simulink model "simul_exp3"  (R2018a)
settings: Solver=VariableStepDiscrete  StartTime=0.0  StopTime=0.2  RelTol=1e-3
libraries: powerlib_meascontrol x12, powerlib x8
settings Model: Creator=PSA LAB  LastModifiedBy=PSA LAB

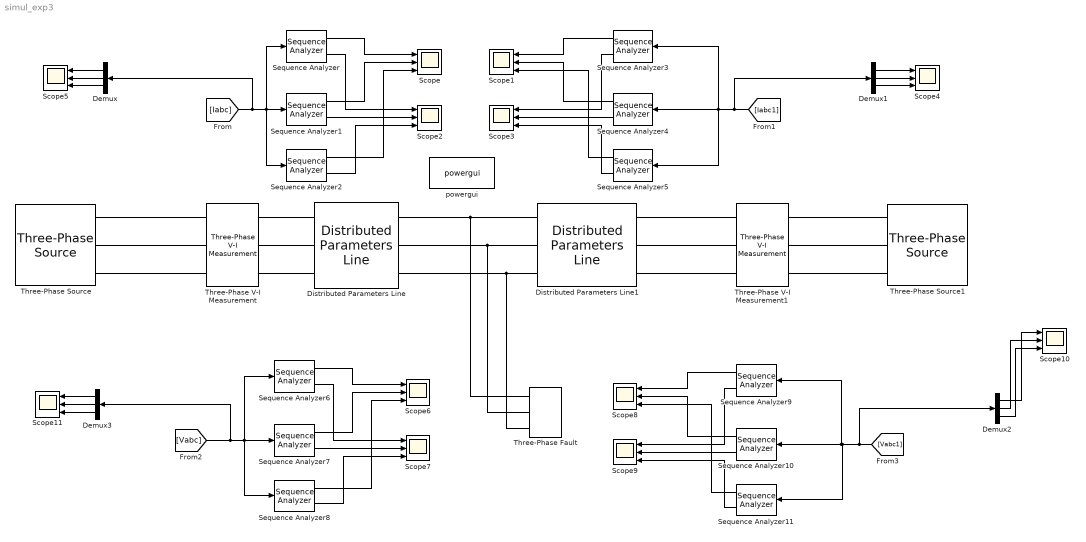
== system simul_exp3 ==
  Demux{,1..3} (4 alike) : Demux  Outputs=3
  Distributed Parameters Line : powerlib/Elements/Distributed Parameters Line  Phases=3  Frequency=50  Resistance=[0.0168 0.242]  Inductance=[0.223 0.724]/(2*pi*50)  Capacitance=[12.74e-9 7.751e-9]  Length=50  x1=[-0.00025 -1.56487866400999e-10 0 0;-0.0002 -1.54369226650682e-10 255080.19880985 -307468.607575482;-0.00015 -1.52212498603565e-10 259878.237181357 -303424.050313729;-0.0001 -1.50018214400022e-10 264612.154486481 -299304.627707794;-5e-05 -1.47786915446847e-10 269280.782701962 -295111.356163562]  x2=[-0.00025 -1.7683899889414e-10 0 0;-0.0002 -1.82309191569534e-10 234319.785127672 -322361.576827908;-0.00015 -1.87734402179861e-10 239354.313253658 -318641.272662729;-0.0001 -1.93113292135579e-10 244329.784284384 -314842.348531452;-5e-05 -1.98444534276079e-10 249244.970596823 -310965.741761762]  x3=[-0.00025 1.20606379414602e-11 0 0;-0.0002 1.20492587104112e-11 -418.457428681975 424.341761235616;-0.00015 1.20349065050724e-11 -425.071075319853 417.716567631808;-0.0001 1.20175848666357e-11 -431.579842030371 410.988308715365;-5e-05 1.1997298068956e-11 -437.982122872735 404.158644583495]  x4=[-0.00025 -1.34129195403542e-11 0 0;-0.0002 -1.33002997678989e-11 2423.35362344846 -3134.39626162489;-0.00015 -1.31843983454925e-11 2472.2876169882 -3095.94519461435;-0.0001 -1.30652438700767e-11 2520.61161055209 -3056.73024945266;-5e-05 -1.29428657412354e-11 2568.31368091779 -3016.76110184075]  x5=0.000211321273641276  V1=[1.455e-10 3.995e+05 3.995e+05;314.2 314.2 314.2;0.5771 0.7081 -0.8627]  V2=[5.043e-10 3.985e+05 3.985e+05;314.2 314.2 314.2;-0.8314 0.6441 -0.9267]  I1=[1.151e-11 596 596;314.2 314.2 314.2;-2.267 -2.348 2.365]  I2=[1.656e-11 3962 3962;314.2 314.2 314.2;0.6614 0.6737 -0.897]  nHarmo=1  Measurements=None
      settings: SourceProductName=Simscape Power Systems
  Distributed Parameters Line1 : powerlib/Elements/Distributed Parameters Line  Phases=3  Frequency=50  Resistance=[0.0168 0.242]  Inductance=[0.223 0.724]/(2*pi*50)  Capacitance=[12.74e-9 7.751e-9]  Length=100  x1=[-0.00045 -1.70021553368224e-10 208305.257615079 -339752.362121545;-0.0004 -1.77191466076833e-10 213616.157671673 -336438.5309367;-0.00035 -1.84317659442561e-10 218874.35113777 -333041.688578584;-0.0003 -1.91398375183826e-10 224078.54063281 -329562.67316722;-0.00025 -1.98431866239969e-10 229227.442100909 -326002.343097605;-0.0002 -2.05416397202318e-10 234319.785127672 -322361.576827908;-0.00015 -2.12350244742368e-10 239354.313253658 -318641.272662729;-0.0001 -2.19231698036993e-10 244329.784284384 -314842.348531452;-5e-05 -2.26059059190562e-10 249244.970596823 -310965.741761762]  x2=[-0.00045 -1.06944269874296e-10 163412.8471615 -363782.763094215;-0.0004 -1.04861400083317e-10 169106.738616573 -361171.106674324;-0.00035 -1.02752657310943e-10 174758.90551429 -358470.33668818;-0.0003 -1.00618561857898e-10 180367.953267046 -355681.119510365;-0.00025 -9.84596402803031e-11 185932.497926236 -352804.143338482;-0.0002 -9.62764252597519e-11 191451.166523731 -349840.118023352;-0.00015 -9.40694554718829e-11 196922.597410631 -346789.774893869;-0.0001 -9.18392754534677e-11 202345.440593236 -343653.866576558;-5e-05 -8.9586435468055e-11 207718.358066135 -340433.166809873]  x3=[-0.00045 -7.36346410085895e-12 -409.538920507377 443.963253695975;-0.0004 -7.37107802688559e-12 -416.461868407682 437.475725275183;-0.00035 -7.3768732497049e-12 -423.282060573609 430.880256265269;-0.0003 -7.38084833943238e-12 -429.997814224796 424.178473999522;-0.00025 -7.38300231527411e-12 -436.607472349517 417.372032042433;-0.0002 -7.38333464576877e-12 -443.109404113535 410.46260978171;-0.00015 -7.3818452489188e-12 -449.502005262476 403.451912013908;-0.0001 -7.37853449221059e-12 -455.783698517661 396.341668523796;-5e-05 -7.3734031925238e-12 -461.952933965275 389.133633657564]  x4=[-0.00045 5.90981358690036e-12 1835.53978451295 -3482.79405347785;-0.0004 5.8270331277052e-12 1890.01868985462 -3453.53298398477;-0.00035 5.74281493527755e-12 1944.03126136552 -3423.41980690421;-0.0003 5.6571797891962e-12 1997.56417225185 -3392.46195221203;-0.00025 5.57014881865206e-12 2050.60421406887 -3360.66705829565;-0.0002 5.48174349723485e-12 2103.13829997991 -3328.04297006936;-0.00015 5.39198563763478e-12 2155.15346798537 -3294.59773703879;-0.0001 5.30089738626064e-12 2206.63688412086 -3260.33961131473;-5e-05 5.20850121777547e-12 2257.57584562381 -3225.27704557708]  x5=0.000422642547282553  V1=[5.043e-10 3.985e+05 3.985e+05;314.2 314.2 314.2;-0.8978 0.5969 -0.9739]  V2=[1.841e-10 3.988e+05 3.988e+05;314.2 314.2 314.2;0.189 0.4691 -1.102]  I1=[3.598e-12 604 604;314.2 314.2 314.2;0.6362 -2.35 2.363]  I2=[5.12e-12 3937 3937;314.2 314.2 314.2;-2.674 0.5319 -1.039]  nHarmo=1  Measurements=None
      settings: SourceProductName=Simscape Power Systems
  Scope{,1..11} (12 alike) : Scope  NumInputPorts=3
  Sequence Analyzer{,3,6,9} (4 alike) : powerlib_meascontrol/Measurements/Sequence Analyzer  Freq=50  n=1  seq=Positive  InInit=[1, 0]  Ts=0
      settings: SourceProductName=Simscape Power Systems  SourceProductBaseCode=PS
  Sequence Analyzer{1,4,7,10} (4 alike) : powerlib_meascontrol/Measurements/Sequence Analyzer  Freq=50  n=1  seq=Negative  InInit=[1, 0]  Ts=0
      settings: SourceProductName=Simscape Power Systems  SourceProductBaseCode=PS
  Sequence Analyzer{2,5,8,11} (4 alike) : powerlib_meascontrol/Measurements/Sequence Analyzer  Freq=50  n=1  seq=Zero  InInit=[1, 0]  Ts=0
      settings: SourceProductName=Simscape Power Systems  SourceProductBaseCode=PS
  Three-Phase V-I Measurement : powerlib/Measurements/Three-Phase V-I Measurement  VoltageMeasurement=phase-to-phase  SetLabelV=on  LabelV=Vabc  Vpu=off  VpuLL=on  CurrentMeasurement=yes  SetLabelI=on  LabelI=Iabc  Ipu=on  Pbase=100e6  Vbase=400e3  OutputType=Complex  PhasorSimulation=off  PSBequivalent=0
  Three-Phase V-I Measurement1 : powerlib/Measurements/Three-Phase V-I Measurement  VoltageMeasurement=phase-to-phase  SetLabelV=on  LabelV=Vabc1  Vpu=off  VpuLL=on  CurrentMeasurement=yes  SetLabelI=on  LabelI=Iabc1  Ipu=on  Pbase=100e6  Vbase=400e3  OutputType=Complex  PhasorSimulation=off  PSBequivalent=0
  Three-Phase Fault : powerlib/Elements/Three-Phase Fault  InitialStates=0  FaultA=on  FaultB=off  FaultC=off  GroundFault=on  SwitchTimes=[40e-3]  External=off  SwitchStatus=NaN  FaultResistance=1  GroundResistance=0.01  SnubberResistance=1e6  SnubberCapacitance=inf  Measurements=None
  Three-Phase Source : powerlib/Electrical Sources/Three-Phase Source  InternalConnection=Yg  VoltagePhases=off  Voltage=400e+3  PhaseAngle=15  Voltage_phases=[25e3 25e3 25e3]/sqrt(3)  PhaseAngles_phases=[0 -120 +120]  Frequency=50  NonIdealSource=on  SpecifyImpedance=off  Resistance=0.256  Inductance=5.248/(2*pi*50)  ShortCircuitLevel=100e6  BaseVoltage=400  XRratio=7  BusType=swing  Pref=10e3  Qref=0  Prefabc=[10e3, 10e3, 10e3]  Qrefabc=[0, 0, 0]  Qmin=-inf  Qmax=inf
  Three-Phase Source1 : powerlib/Electrical Sources/Three-Phase Source  InternalConnection=Yg  VoltagePhases=off  Voltage=400e+3  PhaseAngle=0  Voltage_phases=[25e3 25e3 25e3]/sqrt(3)  PhaseAngles_phases=[0 -120 +120]  Frequency=50  NonIdealSource=on  SpecifyImpedance=off  Resistance=0.384  Inductance=7.04/(2*pi*50)  ShortCircuitLevel=100e6  BaseVoltage=400  XRratio=7  BusType=swing  Pref=10e3  Qref=0  Prefabc=[10e3, 10e3, 10e3]  Qrefabc=[0, 0, 0]  Qmin=-inf  Qmax=inf
  powergui : powerlib/powergui  Priority=1  SimulationMode=Continuous  SampleTime=50e-6  frequency=60  Iterations=50  frequencyindice=50  Pbase=100e6  ErrMax=1e-4  UnitsV=kV  UnitsW=MW  buscounter=0  FunctionMessages=off  echomessages=off  EnableUseOfTLC=off  CurrentSourceSwitches=off  DisableSnubberDevices=off  DisableRonSwitches=off  DisableVfSwitches=off  DisplayEquations=off  SolverType=Tustin/Backward Euler (TBE)  Interpol=off  ExternalGateDelay=off  methode=off  Ts=100  x0status=blocks  SPID=on  SwTol=0  HookPort=off  RestoreLinks=warning  ResistiveCurrentMeasurement=off  Frange=[0:2:500]  Ylog=off  Xlog=on  ShowGrid=off  save=off  variable=ZData  structure=0  ZoomFFT=off  StartTime=0.0  cycles=1  DisplayStyle=1  fundamental=60  FreqAxis=off  MaxFrequency=1000  frequencyindicesteady=1  RmsSteady=1  display=off
  wires:
  Sequence Analyzer/1 -> Scope/1
  Sequence Analyzer1/1 -> Scope/2
  Sequence Analyzer2/1 -> Scope/3
  Sequence Analyzer/2 -> Scope2/1
  Sequence Analyzer1/2 -> Scope2/2
  Sequence Analyzer2/2 -> Scope2/3
  Sequence Analyzer3/1 -> Scope1/1
  Sequence Analyzer4/1 -> Scope1/2
  Sequence Analyzer5/1 -> Scope1/3
  Sequence Analyzer3/2 -> Scope3/1
  Sequence Analyzer4/2 -> Scope3/2
  Sequence Analyzer5/2 -> Scope3/3
  [Iabc] -> Demux/1, Sequence Analyzer/1, Sequence Analyzer2/1, Sequence Analyzer1/1
  [Iabc1] -> Demux1/1, Sequence Analyzer5/1, Sequence Analyzer3/1, Sequence Analyzer4/1
  Demux1/1 -> Scope4/1
  Demux1/2 -> Scope4/2
  Demux1/3 -> Scope4/3
  Demux/1 -> Scope5/1
  Demux/2 -> Scope5/2
  Demux/3 -> Scope5/3
  [Vabc] -> Demux3/1, Sequence Analyzer8/1, Sequence Analyzer6/1, Sequence Analyzer7/1
  Sequence Analyzer6/2 -> Scope7/1
  Sequence Analyzer6/1 -> Scope6/1
  Sequence Analyzer7/2 -> Scope7/2
  Sequence Analyzer8/2 -> Scope7/3
  Sequence Analyzer8/1 -> Scope6/3
  Sequence Analyzer7/1 -> Scope6/2
  Sequence Analyzer10/2 -> Scope9/2
  Sequence Analyzer11/1 -> Scope8/3
  Sequence Analyzer10/1 -> Scope8/2
  Sequence Analyzer9/2 -> Scope9/1
  Sequence Analyzer11/2 -> Scope9/3
  [Vabc1] -> Demux2/1, Sequence Analyzer11/1, Sequence Analyzer9/1, Sequence Analyzer10/1
  Sequence Analyzer9/1 -> Scope8/1
  Demux2/2 -> Scope10/2
  Demux2/1 -> Scope10/1
  Demux2/3 -> Scope10/3
  Demux3/1 -> Scope11/1
  Demux3/2 -> Scope11/2
  Demux3/3 -> Scope11/3
  connections:
  Three-Phase V-I Measurement/RConn1 -- Distributed Parameters Line/LConn1
  Three-Phase V-I Measurement/RConn2 -- Distributed Parameters Line/LConn2
  Three-Phase V-I Measurement/RConn3 -- Distributed Parameters Line/LConn3
  Three-Phase Source/RConn2 -- Three-Phase V-I Measurement/LConn2
  Three-Phase Source/RConn1 -- Three-Phase V-I Measurement/LConn1
  Three-Phase Source/RConn3 -- Three-Phase V-I Measurement/LConn3
  Distributed Parameters Line1/RConn1 -- Three-Phase V-I Measurement1/RConn1
  Distributed Parameters Line1/RConn2 -- Three-Phase V-I Measurement1/RConn2
  Distributed Parameters Line1/RConn3 -- Three-Phase V-I Measurement1/RConn3
  Three-Phase Source1/RConn2 -- Three-Phase V-I Measurement1/LConn2
  Three-Phase Source1/RConn3 -- Three-Phase V-I Measurement1/LConn3
  Three-Phase Source1/RConn1 -- Three-Phase V-I Measurement1/LConn1
  Distributed Parameters Line/RConn1 -- Three-Phase Fault/LConn1 -- Distributed Parameters Line1/LConn1
  Distributed Parameters Line/RConn2 -- Three-Phase Fault/LConn2 -- Distributed Parameters Line1/LConn2
  Distributed Parameters Line/RConn3 -- Three-Phase Fault/LConn3 -- Distributed Parameters Line1/LConn3
